simulink model "test06"  (R2022a)
settings: Solver=FixedStepAuto  StartTime=0  StopTime=5  FixedStep=0.1  RelTol=1e-3
InitFcn:
  | Init_data
values from neighbouring files (symbols this model uses):
  dq0 = 0    [Init_data.m]
  dqm = [0,0,0,0].'    [Init_data.m]
  Kdbf = 5    [Init_data.m]
  Kdmf = diag([10,15,10,15])    [Init_data.m]
  Kibc = 1    [Init_data.m]
  Kimc = diag([1,1,1,1])    [Init_data.m]
  Kimf = diag([2,2,2,2])    [Init_data.m]
  Kpbc = 1    [Init_data.m]
  Kpbf = 10    [Init_data.m]
  Kpmc = diag([1,1,1,1])    [Init_data.m]
  Kpmf = diag([1,1,1,1])    [Init_data.m]
  q0 = 0.3    [Init_data.m]    (also in calc_Mass.m = w0)
  q0_d = 0    [Init_data.m]
  qm = [0.1,0.15,0.25,0.3].'    [Init_data.m]
  qm_d = [0,0,0,0].'    [Init_data.m]
undefined symbols (not defined in the file or in its folder): Kdf, Kif, Kpf
settings Model: Creator=43840  LastModifiedBy=43840

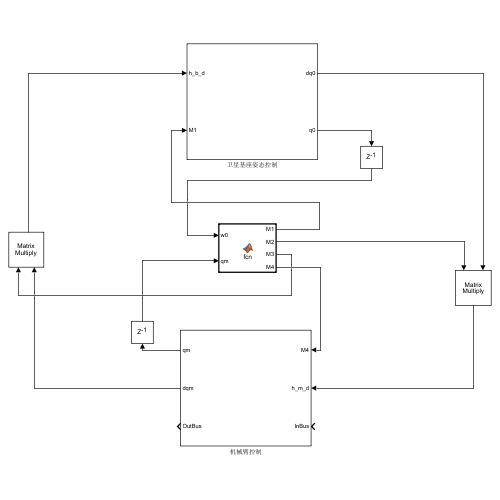
[thumbnail: Simulink's stored preview of the top-level diagram]
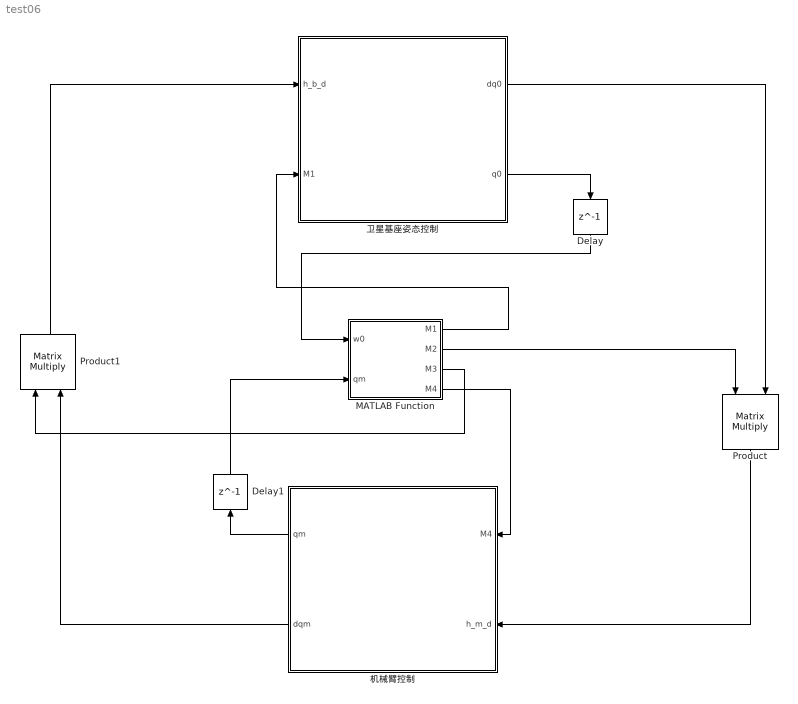
== system test06 ==
  Delay : Delay  DelayLength=1
  Delay1 : Delay  DelayLength=1
  MATLAB Function : MATLAB Function  TreatAsAtomicUnit=on
  Product : Product  Multiplication=Matrix(*)
  Product1 : Product  Multiplication=Matrix(*)
  卫星基座姿态控制 : Subsystem
  机械臂控制 : Subsystem
  wires:
  Product1/1 -> 卫星基座姿态控制/1(h_b_d)
  机械臂控制/2(dqm) -> Product1/2
  Product/1 -> 机械臂控制/2(h_m_d)
  卫星基座姿态控制/1(dq0) -> Product/2
  机械臂控制/1(qm) -> Delay1/1
  卫星基座姿态控制/2(q0) -> Delay/1
  MATLAB Function/1(M1) -> 卫星基座姿态控制/2(M1)
  MATLAB Function/4(M4) -> 机械臂控制/1(M4)
  MATLAB Function/2(M2) -> Product/1
  MATLAB Function/3(M3) -> Product1/1
  Delay/1 -> MATLAB Function/1(w0)
  Delay1/1 -> MATLAB Function/2(qm)

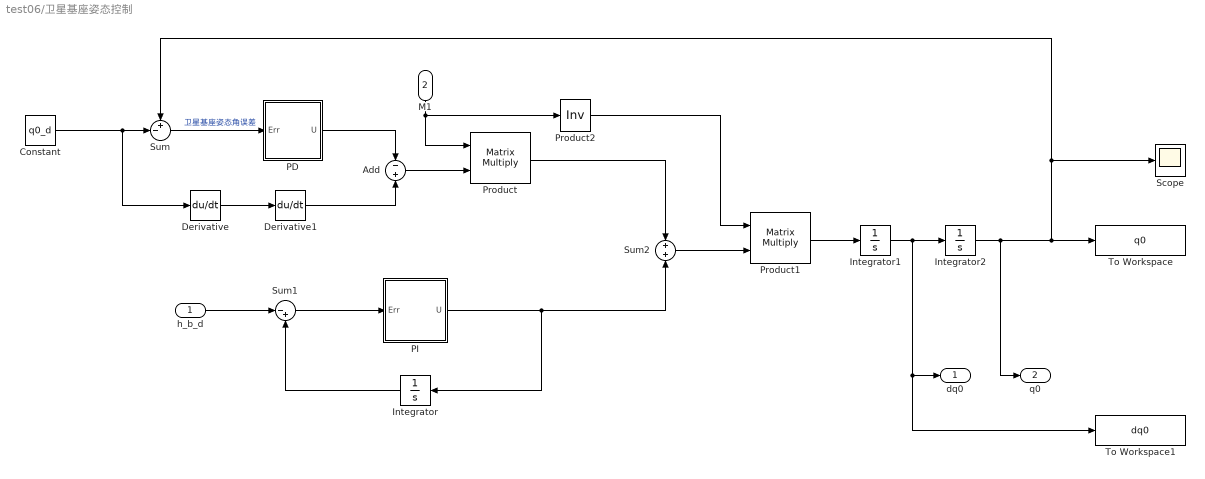
== system test06/卫星基座姿态控制 ==
  h_b_d : Inport
  M1 : Inport  Port=2
  Add : Sum  Inputs=-+
  Constant : Constant  Value=q0_d
  Derivative : Derivative
  Derivative1 : Derivative
  Integrator : Integrator
  Integrator1 : Integrator  InitialCondition=dq0
  Integrator2 : Integrator  InitialCondition=q0
  PD : Subsystem
  PI : Subsystem
  Product : Product  Multiplication=Matrix(*)
  Product1 : Product  Multiplication=Matrix(*)
  Product2 : Product  Inputs=/  Multiplication=Matrix(*)
  Scope : Scope
  Sum : Sum  Inputs=+-|
  Sum1 : Sum  Inputs=|-+
  Sum2 : Sum  Inputs=+|+
  To Workspace : ToWorkspace  VariableName=q0  SampleTime=-1
      settings: Save2DSignal=2-D array (concatenate along first dimension)
  To Workspace1 : ToWorkspace  VariableName=dq0  SampleTime=-1
      settings: Save2DSignal=2-D array (concatenate along first dimension)
  dq0 : Outport
  q0 : Outport  Port=2
  wires:
  Sum/1 -> PD/1(Err)  "卫星基座姿态角误差"
  Integrator/1 -> Sum1/2
  Sum1/1 -> PI/1(Err)
  Derivative/1 -> Derivative1/1
  Product/1 -> Sum2/1
  PD/1(U) -> Add/1
  Add/1 -> Product/2
  PI/1(U) -> Sum2/2, Integrator/1
  h_b_d/1 -> Sum1/1
  Integrator1/1 -> Integrator2/1, To Workspace1/1, dq0/1
  Derivative1/1 -> Add/2
  Constant/1 -> Derivative/1, Sum/2
  Integrator2/1 -> q0/1, To Workspace/1, Scope/1, Sum/1
  M1/1 -> Product2/1, Product/1
  Product2/1 -> Product1/1
  Product1/1 -> Integrator1/1
  Sum2/1 -> Product1/2

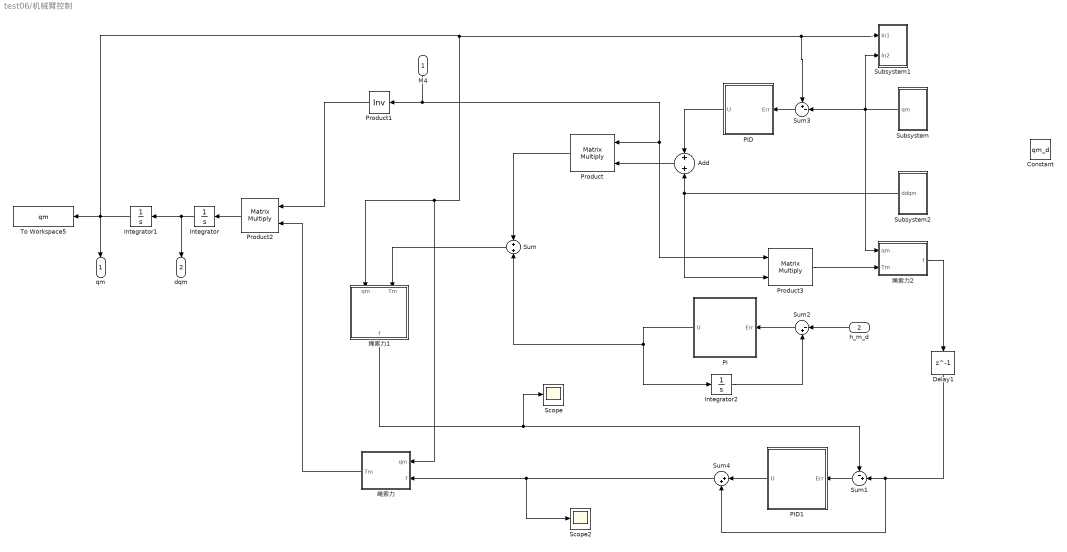
== system test06/机械臂控制 ==
  M4 : Inport
  h_m_d : Inport  Port=2
  Add : Sum
  Constant : Constant  Value=qm_d
  Delay1 : Delay  DelayLength=1
  Integrator : Integrator  InitialCondition=dqm
  Integrator1 : Integrator  InitialCondition=qm
  Integrator2 : Integrator
  PI : Subsystem
  PID : Subsystem
  PID1 : Subsystem
  Product : Product  Multiplication=Matrix(*)
  Product1 : Product  Inputs=/  Multiplication=Matrix(*)
  Product2 : Product  Multiplication=Matrix(*)
  Product3 : Product  Multiplication=Matrix(*)
  Scope : Scope
  Scope2 : Scope
  Subsystem : Subsystem
  Subsystem1 : Subsystem
  Subsystem2 : Subsystem
  Sum : Sum
  Sum1 : Sum  Inputs=-+|
  Sum2 : Sum  Inputs=|-+
  Sum3 : Sum  Inputs=+-|
  Sum4 : Sum  Inputs=|++
  To Workspace5 : ToWorkspace  VariableName=qm  SampleTime=-1
      settings: Save2DSignal=2-D array (concatenate along first dimension)
  绳索力 : MATLAB Function  TreatAsAtomicUnit=on
  绳索力1 : MATLAB Function  TreatAsAtomicUnit=on
  绳索力2 : MATLAB Function  TreatAsAtomicUnit=on
  qm : Outport
  dqm : Outport  Port=2
  wires:
  Integrator2/1 -> Sum2/2
  PI/1(U) -> Sum/2, Integrator2/1
  Sum2/1 -> PI/1(Err)
  Product2/1 -> Integrator/1
  h_m_d/1 -> Sum2/1
  M4/1 -> Product/1, Product3/1, Product1/1
  Integrator/1 -> Integrator1/1, dqm/1
  Product1/1 -> Product2/1
  Subsystem2/1(ddqm) -> Product3/2, Add/2
  Add/1 -> Product/2
  Product/1 -> Sum/1
  Sum3/1 -> PID/1(Err)
  PID/1(U) -> Add/1
  Subsystem/1(qm) -> Sum3/2, 绳索力2/1(qm), Subsystem1/2(In2)
  Integrator1/1 -> Subsystem1/1(In1), Sum3/1, 绳索力/1(qm), 绳索力1/1(qm), To Workspace5/1, qm/1
  Product3/1 -> 绳索力2/2(Tm)
  Sum/1 -> 绳索力1/2(Tm)
  绳索力/1(Tm) -> Product2/2
  绳索力2/1(f) -> Delay1/1
  绳索力1/1(f) -> Scope/1, Sum1/1
  Sum1/1 -> PID1/1(Err)
  PID1/1(U) -> Sum4/1
  Sum4/1 -> Scope2/1, 绳索力/2(f)
  Delay1/1 -> Sum1/2, Sum4/2

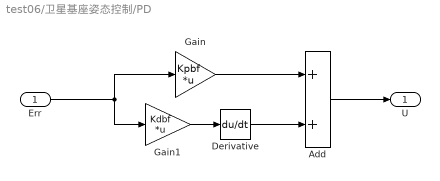
== system test06/卫星基座姿态控制/PD ==
  Err : Inport
  Add : Sum
  Derivative : Derivative
  Gain : Gain  Gain=Kpbf  Multiplication=Matrix(K*u)
  Gain1 : Gain  Gain=Kdbf  Multiplication=Matrix(K*u)
  U : Outport
  wires:
  Err/1 -> Gain1/1, Gain/1
  Gain1/1 -> Derivative/1
  Gain/1 -> Add/1
  Derivative/1 -> Add/2
  Add/1 -> U/1

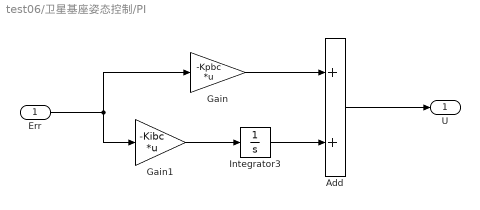
== system test06/卫星基座姿态控制/PI ==
  Err : Inport
  Add : Sum
  Gain : Gain  Gain=-Kpbc  Multiplication=Matrix(K*u)
  Gain1 : Gain  Gain=-Kibc  Multiplication=Matrix(K*u)
  Integrator3 : Integrator
  U : Outport
  wires:
  Gain1/1 -> Integrator3/1
  Add/1 -> U/1
  Gain/1 -> Add/1
  Err/1 -> Gain1/1, Gain/1
  Integrator3/1 -> Add/2

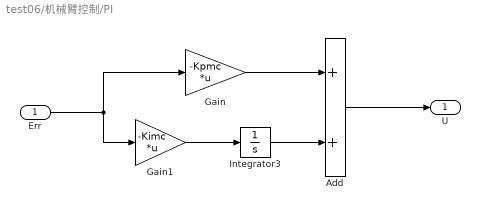
== system test06/机械臂控制/PI ==
  Err : Inport
  Add : Sum
  Gain : Gain  Gain=-Kpmc  Multiplication=Matrix(K*u)
  Gain1 : Gain  Gain=-Kimc  Multiplication=Matrix(K*u)
  Integrator3 : Integrator
  U : Outport
  wires:
  Gain1/1 -> Integrator3/1
  Add/1 -> U/1
  Gain/1 -> Add/1
  Err/1 -> Gain1/1, Gain/1
  Integrator3/1 -> Add/2

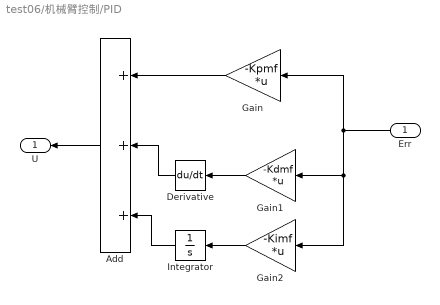
== system test06/机械臂控制/PID ==
  Err : Inport
  Add : Sum  Inputs=+++
  Derivative : Derivative
  Gain : Gain  Gain=-Kpmf  Multiplication=Matrix(K*u)
  Gain1 : Gain  Gain=-Kdmf  Multiplication=Matrix(K*u)
  Gain2 : Gain  Gain=-Kimf  Multiplication=Matrix(K*u)
  Integrator : Integrator
  U : Outport
  wires:
  Add/1 -> U/1
  Derivative/1 -> Add/2
  Gain/1 -> Add/1
  Gain1/1 -> Derivative/1
  Err/1 -> Gain2/1, Gain1/1, Gain/1
  Gain2/1 -> Integrator/1
  Integrator/1 -> Add/3

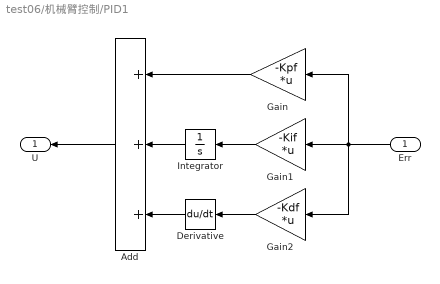
== system test06/机械臂控制/PID1 ==
  Err : Inport
  Add : Sum  Inputs=+++
  Derivative : Derivative
  Gain : Gain  Gain=-Kpf  Multiplication=Matrix(K*u)
  Gain1 : Gain  Gain=-Kif  Multiplication=Matrix(K*u)
  Gain2 : Gain  Gain=-Kdf  Multiplication=Matrix(K*u)
  Integrator : Integrator
  U : Outport
  wires:
  Gain2/1 -> Derivative/1
  Derivative/1 -> Add/3
  Integrator/1 -> Add/2
  Gain1/1 -> Integrator/1
  Add/1 -> U/1
  Gain/1 -> Add/1
  Err/1 -> Gain2/1, Gain1/1, Gain/1

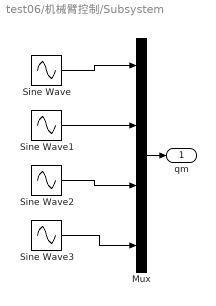
== system test06/机械臂控制/Subsystem ==
  Mux : Mux
  Sine Wave : Sin  Amplitude=0.4  Frequency=0.2  SampleTime=0
  Sine Wave1 : Sin  Amplitude=0.3  Frequency=0.2  SampleTime=0
  Sine Wave2 : Sin  Amplitude=0.2  Frequency=0.2  SampleTime=0
  Sine Wave3 : Sin  Amplitude=0.1  Frequency=0.2  SampleTime=0
  qm : Outport
  wires:
  Sine Wave2/1 -> Mux/3
  Sine Wave1/1 -> Mux/2
  Mux/1 -> qm/1
  Sine Wave3/1 -> Mux/4
  Sine Wave/1 -> Mux/1

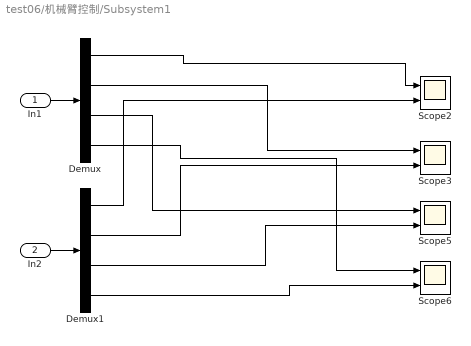
== system test06/机械臂控制/Subsystem1 ==
  In1 : Inport
  In2 : Inport  Port=2
  Demux : Demux
  Demux1 : Demux
  Scope{2..3,5..6} (4 alike) : Scope  NumInputPorts=2
  wires:
  Demux1/1 -> Scope2/2
  Demux/3 -> Scope5/1
  Demux1/2 -> Scope3/2
  Demux1/4 -> Scope6/2
  In2/1 -> Demux1/1
  Demux/2 -> Scope3/1
  Demux1/3 -> Scope5/2
  Demux/4 -> Scope6/1
  Demux/1 -> Scope2/1
  In1/1 -> Demux/1

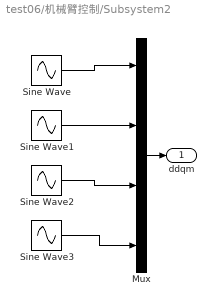
== system test06/机械臂控制/Subsystem2 ==
  Mux : Mux
  Sine Wave{,1..3} (4 alike) : Sin  Amplitude=-0.064*pi^2  Frequency=0.2  Phase=pi/2  SampleTime=0
  ddqm : Outport
  wires:
  Sine Wave/1 -> Mux/1
  Sine Wave3/1 -> Mux/4
  Mux/1 -> ddqm/1
  Sine Wave1/1 -> Mux/2
  Sine Wave2/1 -> Mux/3

== matlab function test06/机械臂控制/绳索力2 ==
  data: qm input; Tm input; f output
function f = fcn(qm,Tm)

coder.extrinsic("calc_J_hat")

f=zeros(8,1);

f=calc_J_hat(qm,Tm);

== matlab function test06/MATLAB Function ==
  data: w0 input; M1 output; qm input; M2 output; M3 output; M4 output
function [M1, M2, M3, M4] = fcn(w0,qm)

coder.extrinsic("calc_Mass")

M1=zeros(1,1);
M2=zeros(4,1);
M3=zeros(1,4);
M4=zeros(4,4);

[M1, M2, M3, M4]=calc_Mass(w0,qm);

== matlab function test06/机械臂控制/绳索力1 ==
  data: qm input; Tm input; f output
function f = fcn(qm,Tm)

coder.extrinsic("calc_J_hat")

f=zeros(8,1);

f=calc_J_hat(qm,Tm);

== matlab function test06/机械臂控制/绳索力 ==
  data: qm input; f input; Tm output
function Tm = fcn(qm,f)

coder.extrinsic("calc_J")

Tm=zeros(4,1);

Tm=calc_J(qm,f);
